simulink model "Simulink_Prelab2_mosalas_setare"  (Simulink 7.1)
settings: Solver=ode23t  StartTime=0.0  StopTime=10.0  RelTol=1e-3
libraries: powerlib x6
settings Model: Creator=Rose  LastModifiedBy=Rose

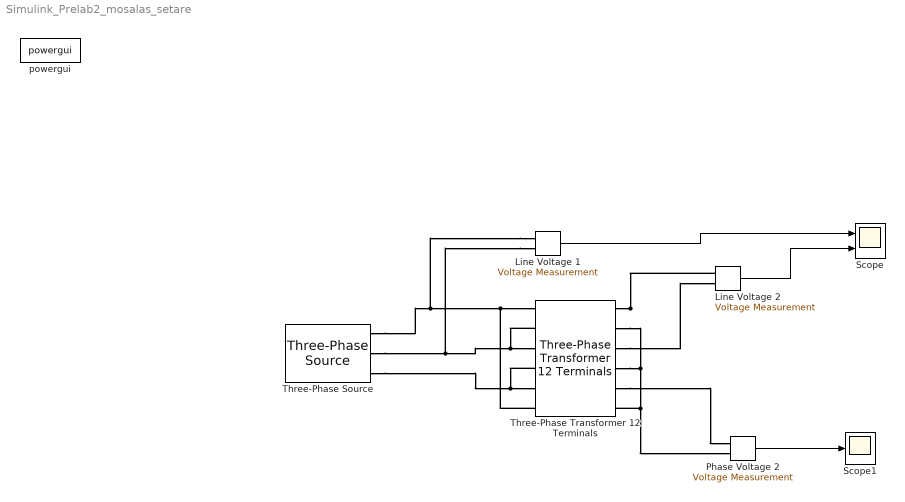
== system Simulink_Prelab2_mosalas_setare ==
  Line Voltage 1 : powerlib/Measurements/Voltage Measurement  DialogController=POWERSYS.PowerSysDialog  SystemSampleTime=-1  PhasorSimulation=off  OutputType=Complex  PSBequivalent=0
  Line Voltage 2 : powerlib/Measurements/Voltage Measurement  DialogController=POWERSYS.PowerSysDialog  SystemSampleTime=-1  PhasorSimulation=off  OutputType=Complex  PSBequivalent=0
  Phase Voltage 2 : powerlib/Measurements/Voltage Measurement  DialogController=POWERSYS.PowerSysDialog  SystemSampleTime=-1  PhasorSimulation=off  OutputType=Complex  PSBequivalent=0
  Scope : Scope  NumInputPorts=2
      settings: YMin=-5~-5  YMax=5~5
  Scope1 : Scope
  Three-Phase Source : powerlib/Electrical Sources/Three-Phase Source  DialogController=POWERSYS.PowerSysDialog  SystemSampleTime=-1  Voltage=10e3*sqrt(3)  PhaseAngle=0  Frequency=60  InternalConnection=Yg  SpecifyImpedance=off  Resistance=0.8929  Inductance=16.58e-3  ShortCircuitLevel=100e6  BaseVoltage=25e3  XRratio=7
  Three-Phase Transformer 12 Terminals : powerlib/Elements/Three-Phase Transformer 12 Terminals  DialogController=POWERSYS.PowerSysDialog  SystemSampleTime=-1  RatedPower=[ 10e6 60 ]  Winding1="[ 10e3 0.002  0.05 ]"  Winding2=[ 25e3 0.002 0.05]  RmXm=[ 200 200 ]
  powergui : powerlib/powergui  SystemSampleTime=-1  SimulationMode=Continuous  SampleTime=50e-6  frequency=60  SPID=off  SwTol=0  Interpol=off  x0status=blocks  echomessages=off  HookPort=off  FunctionMessages=off  EnableUseOfTLC=off  RestoreLinks=warning  frequencyindice=60  Frange=[0:2:500]  Ylog=off  Xlog=on  ShowGrid=off  save=off  variable=ZData  ZoomFFT=on  StartTime=0.0  cycles=1  DisplayStyle=1  fundamental=60  FreqAxis=off  MaxFrequency=1000  frequencyindicesteady=1  RmsSteady=1  display=off  Ts=0  methode=off
  wires:
  Line Voltage 1/1 -> Scope/1
  Line Voltage 2/1 -> Scope/2
  Phase Voltage 2/1 -> Scope1/1
  connections:
  Line Voltage 2/LConn1 -- Three-Phase Transformer 12 Terminals/RConn1
  Line Voltage 1/LConn2 -- Three-Phase Source/RConn2 -- Three-Phase Transformer 12 Terminals/LConn2 -- Three-Phase Transformer 12 Terminals/LConn3
  Three-Phase Source/RConn3 -- Three-Phase Transformer 12 Terminals/LConn4 -- Three-Phase Transformer 12 Terminals/LConn5
  Line Voltage 1/LConn1 -- Three-Phase Source/RConn1 -- Three-Phase Transformer 12 Terminals/LConn6 -- Three-Phase Transformer 12 Terminals/LConn1
  Three-Phase Transformer 12 Terminals/RConn2 -- Three-Phase Transformer 12 Terminals/RConn4 -- Three-Phase Transformer 12 Terminals/RConn6 -- Phase Voltage 2/LConn2
  Three-Phase Transformer 12 Terminals/RConn3 -- Line Voltage 2/LConn2
  Three-Phase Transformer 12 Terminals/RConn5 -- Phase Voltage 2/LConn1
